simulink library "library_plc2simulink"  (R2017b)
settings: Solver=VariableStepAuto  StartTime=0.0  StopTime=10.0  RelTol=1e-3
libraries: simulink x2
settings Model: Creator=Moritz  LastModifiedBy=Moritz
settings DataIOCC: ReturnWorkspaceOutputs=on
settings SFSimCC: SimUseLocalCustomCode=on
settings RTWCC: RTWUseLocalCustomCode=on

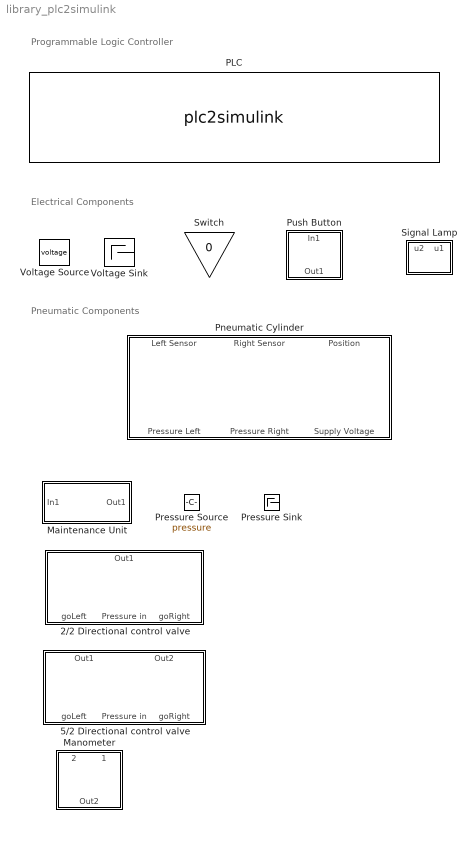
== system library_plc2simulink ==
  note: Programmable Logic Controller
  note: Electrical Components
  note: Pneumatic Components
  2/2 Directional control valve : Subsystem  mask{updateIcon=0.1, state=0}
      mask prompts: updateIcon "Icon Update Time (s):"
      mask init:
      | set_param(gcb,'MaskHideContents','on');
      mask Display:
      | stateValue = strcmpi(get_param(gcb(), 'state'), '1');
      | bigBlockWidth = 0.25;
      | smallBlockWidth = 0.1;
      | 
      | top = 0.85;
      | bottom = 0.3;
      | middle = bottom+(top-bottom)/2;
      | 
      | if ~stateValue
      |     x0=0;
      | else
      |     x0=bigBlockWidth;
      | end
      | 
      | %B1
      | plot(x0+smallBlockWidth*[0,0,1,1,0],[bottom,middle,middle,bottom,bottom]);
      | plot(x0+smallBlockWidth*[1/5,4/5], [bottom, middle]);
      | %B2
      | plot(x0+smallBlockWidth+bigBlockWidth*[0,0,1,1,0],[bottom,top,top,bottom,bottom]);
      | plot(x0+smallBlockWidth+bigBlockWidth*0.5*ones(1,2), [bottom, top]);
      | patch(x0+smallBlockWidth+bigBlockWidth*[0.4,0.5,0.6], top-(top-bottom)/5*[1,0,1]);
      | 
      | %B3
      | plot(x0+smallBlockWidth+bigBlockWidth+bigBlockWidth*[0,0,1,1,0],[bottom,top,top,bottom,bottom]);
      | plot(x0+smallBlockWidth+bigBlockWidth+bigBlockWidth*0.5*ones(1,2), [bottom, bottom+(top-bottom)/5]);
      | plot(x0+smallBlockWidth+bigBlockWidth+bigBlockWidth*0.5*ones(1,2), [top, top-(top-bottom)/5]);
      | plot(x0+smallBlockWidth+bigBlockWidth+bigBlockWidth*0.5+bigBlockWidth/8*[-1,1], top-(top-bottom)/5*ones(1,2));
      | plot(x0+smallBlockWidth+bigBlockWidth+bigBlockWidth*0.5+bigBlockWidth/8*[-1,1], bottom+(top-bottom)/5*ones(1,2));
      | 
      | %B4
      | plot(x0+smallBlockWidth+2*bigBlockWidth+smallBlockWidth*[0,0,1,1,0],[bottom,middle,middle,bottom,bottom]);
      | plot(x0+smallBlockWidth+2*bigBlockWidth+smallBlockWidth*[4/5,1/5], [bottom, middle]);
      | 
      | % Ports
      | port_label('input', 1, 'Ma');
      | port_label('input', 3, 'Mb');
      | 
      | % port connections
      | blockPos = get_param(gcb, 'Position');
      | blockWidthAbs = blockPos(3)-blockPos(1);
      | blockPosXAbs = blockPos(1);
      | ports = get_param(gcb(), 'PortHandles');
      | 
      | pressureIn = ports.Inport(2);
      | pressureInPos = get_param(pressureIn, 'Position');
      | pressureInX = (pressureInPos(1)-blockPosXAbs)/blockWidthAbs;
      | plot(pressureInX*ones(1,2), [0,bottom/2]);
      | plot(smallBlockWidth+bigBlockWidth*1.5*ones(1,2), [bottom/2, bottom]);
      | plot([pressureInX,smallBlockWidth+bigBlockWidth*1.5], bottom/2*ones(1,2));
      | 
      | pressureOut1 = ports.Outport(1);
      | pressureOut1Pos = get_param(pressureOut1, 'Position');
      | pressureOut1X = (pressureOut1Pos(1)-blockPosXAbs)/blockWidthAbs;
      | plot(pressureOut1X*ones(1,2), [1,1-(1-top)/2]);
      | plot(smallBlockWidth+bigBlockWidth*1.5*ones(1,2), [top,1-(1-top)/2]);
      | plot([pressureOut1X,smallBlockWidth+bigBlockWidth*1.5], (1-(1-top)/2)*ones(1,2));
  5/2 Directional control valve : Subsystem  mask{updateIcon=0.1, state=0}
      mask prompts: updateIcon "Update Icon Time (s):"
      mask init:
      | set_param(gcb,'MaskHideContents','on');
      mask Display:
      | stateValue = strcmpi(get_param(gcb(), 'state'), '1');
      | bigBlockWidth = 0.25;
      | smallBlockWidth = 0.1;
      | 
      | top = 0.85;
      | bottom = 0.3;
      | middle = bottom+(top-bottom)/2;
      | 
      | if ~stateValue
      |     x0=0;
      | else
      |     x0=bigBlockWidth;
      | end
      | 
      | %B1
      | plot(x0+smallBlockWidth*[0,0,1,1,0],[bottom,middle,middle,bottom,bottom]);
      | plot(x0+smallBlockWidth*[1/5,4/5], [bottom, middle]);
      | %B2
      | plot(x0+smallBlockWidth+bigBlockWidth*[0,0,1,1,0],[bottom,top,top,bottom,bottom]);
      | plot(x0+smallBlockWidth+bigBlockWidth*[0.5,0.25], [bottom, top]);
      | patch(x0+smallBlockWidth+bigBlockWidth*[0.19,0.29,0.39], top-(top-bottom)/5*[1,0,1]);
      | plot(x0+smallBlockWidth+bigBlockWidth*[0.75,0.75], [bottom, top]);
      | patch(x0+smallBlockWidth+bigBlockWidth*[0.65,0.75,0.85], bottom+(top-bottom)/5*[1,0,1]);
      | plot(x0+smallBlockWidth+bigBlockWidth*0.25*ones(1,2), [bottom, bottom+(top-bottom)/5]);
      | plot(x0+smallBlockWidth+bigBlockWidth*0.25+bigBlockWidth/8*[-1,1], bottom+(top-bottom)/5*ones(1,2));
      | 
      | %B3
      | plot(x0+smallBlockWidth+bigBlockWidth+bigBlockWidth*[0,0,1,1,0],[bottom,top,top,bottom,bottom]);
      | plot(x0+smallBlockWidth+bigBlockWidth+bigBlockWidth*[0.5,0.75], [bottom, top]);
      | patch(x0+smallBlockWidth+bigBlockWidth+bigBlockWidth*[0.63,0.73,0.83], top-(top-bottom)/5*[1,0,1]);
      | plot(x0+smallBlockWidth+bigBlockWidth+bigBlockWidth*[0.25,0.25], [bottom, top]);
      | patch(x0+smallBlockWidth+bigBlockWidth+bigBlockWidth*[0.15,0.25,0.35], bottom+(top-bottom)/5*[1,0,1]);
      | plot(x0+smallBlockWidth+bigBlockWidth+bigBlockWidth*0.75*ones(1,2), [bottom, bottom+(top-bottom)/5]);
      | plot(x0+smallBlockWidth+bigBlockWidth+bigBlockWidth*0.75+bigBlockWidth/8*[-1,1], bottom+(top-bottom)/5*ones(1,2));
      | 
      | %B4
      | plot(x0+smallBlockWidth+2*bigBlockWidth+smallBlockWidth*[0,0,1,1,0],[bottom,middle,middle,bottom,bottom]);
      | plot(x0+smallBlockWidth+2*bigBlockWidth+smallBlockWidth*[4/5,1/5], [bottom, middle]);
      | 
      | % ventiles
      | plot(smallBlockWidth+bigBlockWidth+bigBlockWidth*0.25+bigBlockWidth/8*[-1,0,1], [bottom, bottom-0.1,bottom])
      | plot(smallBlockWidth+bigBlockWidth+bigBlockWidth*0.75+bigBlockWidth/8*[-1,0,1], [bottom, bottom-0.1,bottom])
      | 
      | % Port labels
      | port_label('input', 1, 'Ma');
      | port_label('input', 3, 'Mb');
      | 
      | % port connections
      | blockPos = get_param(gcb, 'Position');
      | blockWidthAbs = blockPos(3)-blockPos(1);
      | blockPosXAbs = blockPos(1);
      | ports = get_param(gcb(), 'PortHandles');
      | 
      | pressureIn = ports.Inport(2);
      | pressureInPos = get_param(pressureIn, 'Position');
      | pressureInX = (pressureInPos(1)-blockPosXAbs)/blockWidthAbs;
      | plot(pressureInX*ones(1,2), [0,bottom/2]);
      | plot(smallBlockWidth+bigBlockWidth*1.5*ones(1,2), [bottom/2, bottom]);
      | plot([pressureInX,smallBlockWidth+bigBlockWidth*1.5], bottom/2*ones(1,2));
      | 
      | pressureOut1 = ports.Outport(1);
      | pressureOut1Pos = get_param(pressureOut1, 'Position');
      | pressureOut1X = (pressureOut1Pos(1)-blockPosXAbs)/blockWidthAbs;
      | plot(pressureOut1X*ones(1,2), [1,1-(1-top)/2]);
      | plot(smallBlockWidth+bigBlockWidth*1.25*ones(1,2), [top,1-(1-top)/2]);
      | plot([pressureOut1X,smallBlockWidth+bigBlockWidth*1.25], (1-(1-top)/2)*ones(1,2));
      | 
      | pressureOut2 = ports.Outport(2);
      | pressureOut2Pos = get_param(pressureOut2, 'Position');
      | pressureOut2X = (pressureOut2Pos(1)-blockPosXAbs)/blockWidthAbs;
      | plot(pressureOut2X*ones(1,2), [1,1-(1-top)/2]);
      | plot(smallBlockWidth+bigBlockWidth*1.75*ones(1,2), [top,1-(1-top)/2]);
      | plot([pressureOut2X,smallBlockWidth+bigBlockWidth*1.75], (1-(1-top)/2)*ones(1,2));
  Maintenance Unit : Subsystem  mask{pressure=1}
      mask prompts: pressure "Pressure (MPa):"
      mask init:
      | set_param(gcb,'MaskHideContents','on');
      mask DialogControl DescGroupVar Prompt: Maintenance Unit
      mask DialogControl DescTextVar Prompt: A pneumatic maintenance unit.
      mask Display:
      | % Get block parameters
      | pos = get_param(gcb, 'Position');
      | width = pos(3)-pos(1);
      | height = pos(4)-pos(2);
      | 
      | % plot box
      | plot([1,1,width-1,width-1,1,1], [1,height-1,height-1,1,1,height-1]);
      | 
      | % plot circle
      | radius = min(floor([width*2/5, height*2/5]))-1;
      | x = floor(width/2  + radius*sin(0:2*pi/50:2*pi));
      | y = floor(height/2 + radius*cos(0:2*pi/50:2*pi));
      | plot(x,y);
      | % plot arrow
      | arrowOuterRadius = 0.7*radius;
      | arrowInnerRadius = 0.2*radius;
      | dPi = pi/4;
      | plot(floor(width/2+arrowOuterRadius*sin(pi/4)*[1,-1]), floor(height/2+arrowOuterRadius*sin(pi/4)*[-1,1]));
      | patch(floor(width/2-[arrowOuterRadius*sin(pi/4),...
      |     arrowInnerRadius*sin(pi/4+dPi),...
      |     arrowInnerRadius*sin(pi/4-dPi)]),...
      |     floor(height/2+[arrowOuterRadius*cos(pi/4),...
      |     arrowInnerRadius*cos(pi/4+dPi),...
      |     arrowInnerRadius*cos(pi/4-dPi)]));
      | 
      | % plot filter
      | borderDash = 0.35;
      | numDash = 4;
      | dashHeight = (height-2)/(numDash+(numDash-1)*borderDash);
      | for i=0:numDash-1
      |     lineStart = 1 + i * dashHeight * (1+borderDash);
      |     plot(width/8*ones(1,2), [lineStart, lineStart+dashHeight]);
      | end
      | plot(width*7/8*ones(1,2), [height*3/4, height-1]);
  "Manometer " : Subsystem  mask{stateOn=0, updateIcon=0.1, actPressure=0.3}
      mask prompts: stateOn "State"; updateIcon "Icon Update Time (s):"; actPressure "Activation Pressure (MPa):"
      mask init:
      | set_param(gcb,'MaskHideContents','on');
      mask DialogControl DescGroupVar Prompt: Manometer
      mask DialogControl DescTextVar Prompt: Electrical contact is closed when pressure exceeds activation pressure.
      mask Display:
      | % Get block parameters
      | active = str2double(get_param(gcb, 'StateOn')) ~= 0;
      | pos = get_param(gcb, 'Position');
      | width = pos(3)-pos(1);
      | height = pos(4)-pos(2);
      | y0Abs = pos(1);
      | ports = get_param(gcb(), 'PortHandles');
      | pressureIn = ports.Inport(1);
      | pressureInPos = get_param(pressureIn, 'Position');
      | pressureInX = (pressureInPos(1)-y0Abs)/width;
      | powerIn = ports.Inport(2);
      | powerInPos = get_param(powerIn, 'Position');
      | powerInY = (powerInPos(1)-y0Abs)/width;
      | powerOut = ports.Outport(1);
      | powerOutPos = get_param(powerOut, 'Position');
      | powerOutY = (powerOutPos(1)-y0Abs)/width;
      | 
      | radius = 0.5;
      | xStart =radius/2;
      | xEnd = 1-radius/2;
      | yStart =  powerInY;
      | yEnd = height;
      | plot([0,xStart], powerInY*ones(1,2))
      | plot([xEnd,0.95], powerInY*ones(1,2))
      | plot(0.95*ones(1,2), [powerInY,powerOutY]);
      | plot([0.95,1], powerOutY*ones(1,2))
      | lineX = 1/2;
      | if active
      |     plot([xStart,xEnd+0.02], [yStart,yStart+radius/6]);
      |     plot(xEnd*ones(1,2), [yStart, yStart+radius/6+0.02])
      |     lineYStart = yStart+radius/12;
      |     lineYEnd = pressureInX;
      | else
      |     plot([xStart,xEnd], [yStart,yStart+radius/2]);
      |     lineYStart = yStart+radius/4;
      |     lineYEnd = pressureInX;
      | end
      | 
      | color('blue')
      | borderDash = 0.35;
      | numDash = 3;
      | dashHeight = (lineYEnd-lineYStart)/(numDash+(numDash-1)*borderDash);
      | for i=0:numDash-1
      |     lineStart = lineYStart + i * dashHeight * (1+borderDash);
      |     plot(lineX*ones(1,2), [lineStart, lineStart+dashHeight]);
      | end
      | borderDash = 0.35;
      | numDash = 3;
      | dashHeight = (lineX-0)/(numDash+(numDash-1)*borderDash);
      | for i=0:numDash-1
      |     lineStart = 0 + i * dashHeight * (1+borderDash);
      |     plot([lineStart, lineStart+dashHeight],lineYEnd*ones(1,2));
      | end
      | %port_label('input', 1, 'P')
  PLC : S-Function  FunctionName=plc2simulink  Parameters=instanceName, supplyVoltage,numInputs, numOutputs, timeStep,1  SFunctionDeploymentMode=off  EnableBusSupport=off  mask{instanceName=PLC1, numInputs=8, numOutputs=8, timeStep=0.05, externalSupplyVoltage=on}
      mask prompts: instanceName "PLC Instance Name"; numInputs "Number of Inputs:"; numOutputs "Number of Outputs:"; timeStep "Communication Update Time (s):"; externalSupplyVoltage "External Supply Voltage"
      mask init:
      | % Process parameters
      | if strcmpi(externalSupplyVoltage, 'on')
      |     supplyVoltage = 1.0;
      | else
      |     supplyVoltage = 0.0;
      | end
      | 
      | % Update SPS block
      | Simulink.Block.eval(gcb());
      mask DialogControl DescGroupVar Prompt: PLC Connection
      mask DialogControl DescTextVar Prompt: Connection to a PLC simulated via PLCSim Advanced.
      mask Display:
      | % Get parameters
      | numInputs = str2num(get_param(gcb(), 'numInputs'));
      | numOutputs = str2num(get_param(gcb(), 'numOutputs'));
      | externalSupplyVoltage = strcmpi(get_param(gcb(), 'externalSupplyVoltage'), 'on');
      | orientationParam = get_param(gcb,'Orientation');
      | rotated = strcmpi(orientationParam, 'up') || strcmpi(orientationParam, 'down');
      | instanceName = get_param(gcb,'instanceName');
      | 
      | % Set input port labels
      | if externalSupplyVoltage
      |     port_label('input',1,'L+');
      | end
      | for i=1:numInputs
      |     if externalSupplyVoltage
      |         idx = i+1;
      |     else
      |         idx = i;
      |     end
      |     port_label('input',idx,sprintf('I%g.%g', floor((i-1)/8), mod((i-1),8)))
      | end
      | 
      | % Set output port labels
      | if externalSupplyVoltage
      |     port_label('output',1,'L0');
      | end
      | for i=1:numOutputs
      |     if externalSupplyVoltage
      |         idx = i+1;
      |     else
      |         idx = i;
      |     end
      |     port_label('output',idx,sprintf('Q%g.%g', floor((i-1)/8), mod((i-1),8)))
      | end
      | % paint icon
      | %plot([0,1,1,0,0], [0,0,1,1,0]);
      | if ~rotated
      |     plot(0.25*ones(1,2), [0,1])
      |     plot(0.75*ones(1,2), [0,1])
      | else
      |     plot([0,1], 0.3*ones(1,2))
      |     plot([0,1], 0.7*ones(1,2))
      | end
      | text(0.5,0.5, instanceName, 'horizontalAlignment', 'center', 'verticalAlignment', 'middle');
  Pneumatic Cylinder : Subsystem  mask{minPos=0, maxPos=100, pistonSpeed=5, currentPos=0, updateIcon=0.1}
      mask prompts: minPos "Minimal Position (cm):"; maxPos "Maximal Position (cm):"; pistonSpeed "Piston Speed (cm/s/MPa):"; currentPos "Position (cm):"; updateIcon "Update Icon (s):"
      mask init:
      | set_param(gcb,'MaskHideContents','on');
      mask DialogControl DescGroupVar Prompt: Double-acting cylinder
      mask DialogControl DescTextVar Prompt: A double acting pneumatic cylinder.
      mask Display:
      | % Calculate relative position of piston
      | pos = str2double(get_param(gcb(), 'currentPos'));
      | maxPos = str2double(get_param(gcb(), 'maxPos'));
      | minPos = str2double(get_param(gcb(), 'minPos'));
      | relPos = (pos-minPos)/(maxPos-minPos);
      | 
      | % y-coordinates of drawn elements
      | bottomWall = 0.1;
      | wallHeight = 0.65;
      | pistonSmallBlockHeight = 0.4;
      | stickHeight = 0.16;
      | magnetHeight = 0.36;
      | magnetInnerHeight = 0.16;
      | 
      | topWall = bottomWall+wallHeight;
      | pistonSmallBlockBottom = bottomWall+(wallHeight-pistonSmallBlockHeight)/2;
      | pistonSmallBlockTop = pistonSmallBlockBottom+pistonSmallBlockHeight;
      | stickBottom = bottomWall+(wallHeight-stickHeight)/2;
      | stickTop = stickBottom+stickHeight;
      | magnetBottom = bottomWall+(wallHeight-magnetHeight)/2;
      | magnetTop = magnetBottom+magnetHeight;
      | magnetInnerBottom = bottomWall+(wallHeight-magnetInnerHeight)/2;
      | magnetInnerTop = magnetInnerBottom+magnetInnerHeight;
      | 
      | % x coordinate of drawn elements
      | stickWidth = 0.45;
      | pistonMainBlockWidth = 0.1;
      | pistonSmallBlockWidth = 0.03;
      | wallMargin = 0.015;
      | leftWall = 0;
      | pistonXMin = leftWall+wallMargin;
      | pistonXMax = 1-(pistonMainBlockWidth + 2*pistonSmallBlockWidth+stickWidth);
      | pistonX = relPos * (pistonXMax-pistonXMin)+pistonXMin;
      | rightWall = pistonXMax + pistonMainBlockWidth + 2*pistonSmallBlockWidth+wallMargin;
      | 
      | 
      | % Wall
      | plot(leftWall*ones(1,2), [bottomWall,topWall]);
      | plot([leftWall,rightWall], bottomWall*ones(1,2));
      | plot([leftWall,rightWall], topWall*ones(1,2));
      | plot(rightWall*ones(1,2), [bottomWall,stickBottom]);
      | plot(rightWall*ones(1,2), [stickTop,topWall]);
      | % piston block
      | plot(pistonX+[0,pistonSmallBlockWidth, pistonSmallBlockWidth, 0, 0], [pistonSmallBlockBottom,pistonSmallBlockBottom,pistonSmallBlockTop,pistonSmallBlockTop, pistonSmallBlockBottom]);
      | plot(pistonX+pistonSmallBlockWidth+[0,pistonMainBlockWidth, pistonMainBlockWidth, 0, 0], [bottomWall,bottomWall,topWall,topWall, bottomWall]);
      | plot(pistonX+pistonSmallBlockWidth+pistonMainBlockWidth+[0,pistonSmallBlockWidth, pistonSmallBlockWidth, 0, 0], [pistonSmallBlockBottom,pistonSmallBlockBottom,pistonSmallBlockTop,pistonSmallBlockTop, pistonSmallBlockBottom]);
      | % magnet
      | quarter = pistonMainBlockWidth/4;
      | patch(pistonX+pistonSmallBlockWidth+quarter+quarter*[0, 2,2,1,1,2,2,0],[magnetTop,magnetTop,magnetInnerTop,magnetInnerTop,magnetInnerBottom,magnetInnerBottom,magnetBottom,magnetBottom])
      | % stick
      | plot(pistonX+2*pistonSmallBlockWidth+pistonMainBlockWidth+[0,stickWidth, stickWidth, 0, 0], [stickBottom,stickBottom,stickTop,stickTop, stickBottom]);
      | 
      | % ports
      | port_label('input', 3, 'L+');
      | port_label('output', 1, 'BGa');
      | port_label('output', 2, 'BGb');
      | port_label('output', 3, 'pos');
      | 
      | % port connections
      | blockPos = get_param(gcb, 'Position');
      | blockWidthAbs = blockPos(3)-blockPos(1);
      | blockPosXAbs = blockPos(1);
      | ports = get_param(gcb(), 'PortHandles');
      | 
      | pressureIn1 = ports.Inport(1);
      | pressureInPos1 = get_param(pressureIn1, 'Position');
      | pressureInX1 = (pressureInPos1(1)-blockPosXAbs)/blockWidthAbs;
      | plot(pressureInX1*ones(1,2), [0,bottomWall/2]);
      | plot((leftWall+2*wallMargin)*ones(1,2), [bottomWall/2, bottomWall]);
      | plot([pressureInX1,leftWall+2*wallMargin], bottomWall/2*ones(1,2));
      | 
      | pressureIn2 = ports.Inport(2);
      | pressureInPos2 = get_param(pressureIn2, 'Position');
      | pressureInX1 = (pressureInPos2(1)-blockPosXAbs)/blockWidthAbs;
      | plot(pressureInX1*ones(1,2), [0,bottomWall/2]);
      | plot((rightWall-2*wallMargin)*ones(1,2), [bottomWall/2, bottomWall]);
      | plot([pressureInX1,rightWall-2*wallMargin], bottomWall/2*ones(1,2));
  Pressure Sink : Terminator
      mask Display: plot([0,1,1,0],[0.5,0,1,0.5]);
  Pressure Source : Constant  Value=pressure  mask{pressure=5}
      mask prompts: pressure "Pressure (MPa):"
      mask DialogControl DescGroupVar Prompt: Pressure Source
      mask DialogControl DescTextVar Prompt: Pneumatic pressure source.
      mask Display: plot([1,0,0,1],[0.5,0,1,0.5]);
  Push Button : Subsystem  mask{deactTime=1, StateOn=0}
      mask prompts: deactTime "Time until automatic deactivation (s):"; StateOn "State (0/1):"
      mask init:
      | set_param(gcb,'MaskHideContents','on');
      settings: OpenFcn=|
      | if str2double(get_param(gcb, 'StateOn')) ==0
      |   set_param(gcb, 'StateOn', '1');
      | end
      mask Display:
      | % Get block parameters
      | active = str2double(get_param(gcb, 'StateOn')) ~= 0;
      | pos = get_param(gcb, 'Position');
      | width = pos(3)-pos(1);
      | height = pos(4)-pos(2);
      | radius = min(floor(height/2), width-4);
      | 
      | xStart = floor((width-radius)/2);
      | xEnd = ceil(width-(width-radius)/2);
      | yStart = floor(height/2);
      | yEnd = height;
      | 
      | plot([0,xStart], yStart*ones(1,2))
      | plot([xEnd,width], yStart*ones(1,2))
      | 
      | lineX = floor(width/2);
      | if active
      |     plot([xStart,xEnd+2], [yStart,yStart+floor(radius/6)]);
      |     plot(xEnd*ones(1,2), [yStart, yStart+floor(radius/6)+2])
      |     lineYStart = yStart+floor(radius/12);
      |     lineYEnd = height-floor(radius/4);
      | else
      |     plot([xStart,xEnd], [yStart,yStart+floor(radius/2)]);
      |     lineYStart = yStart+floor(radius/4);
      |     lineYEnd = height;
      | end
      | 
      | borderDash = 0.35;
      | numDash = 3;
      | dashHeight = (lineYEnd-lineYStart)/(numDash+(numDash-1)*borderDash);
      | for i=0:numDash-1
      |     lineStart = lineYStart + i * dashHeight * (1+borderDash);
      |     plot(lineX*ones(1,2), [lineStart, lineStart+dashHeight]);
      | end
      | plot(lineX+ceil(dashHeight/2)*[-1,1], lineYEnd*ones(1,2));
  Signal Lamp : Subsystem  mask{Value=off, updateTime=0.1, colorOn=[0.2,1,0.2], colorOff=[1,1,1]}
      mask prompts: Value "State:"; updateTime "Update Time (s):"; colorOn "Color when ON:"; colorOff "Color when OFF:"
      mask init:
      | set_param(gcb,'MaskHideContents','on')
      mask TypeOptions Value: off | on
      mask DialogControl DescGroupVar Prompt: Signal Lamp
      mask DialogControl DescTextVar Prompt: Signal lamp which switches to ON if its two inputs are different.
      mask Display:
      | % Get block parameters
      | pos = get_param(gcb, 'Position');
      | width = pos(3)-pos(1);
      | height = pos(4)-pos(2);
      | radius = min(floor([width/2, height/2]))-1;
      | 
      | x = floor(width/2  + radius*sin(0:2*pi/50:2*pi));
      | y = floor(height/2 + radius*cos(0:2*pi/50:2*pi));
      | 
      | if strcmpi(get_param(gcb, 'Value'), 'on');
      |     colorLight = eval(get_param(gcb, 'colorOn'));
      | else
      |     colorLight = eval(get_param(gcb, 'colorOff'));
      | end
      | patch(x,y, colorLight);
      | color('black');
      | plot(x-1,y);
      | xStart = 0.5-0.45*sin(pi/4);
      | plot(floor(width/2+radius*sin(pi/4)*[1,-1]), floor(height/2+radius*sin(pi/4)*[1,-1]));
      | plot(floor(width/2+radius*sin(pi/4)*[1,-1]), floor(height/2+radius*sin(pi/4)*[-1,1]));
      | return;
  Switch : Gain  Gain=0
      settings: OpenFcn=|
      | if str2double(get_param(gcb, 'Gain')) ~=0
      |   set_param(gcb, 'Gain', '0');
      | else
      |   set_param(gcb, 'Gain', '1');
      | end
      mask Display:
      | % Get block parameters
      | active = str2double(get_param(gcb, 'Gain')) ~= 0;
      | pos = get_param(gcb, 'Position');
      | width = pos(3)-pos(1);
      | height = pos(4)-pos(2);
      | radius = min(floor(height/2), width-4);
      | 
      | xStart = floor((width-radius)/2);
      | xEnd = ceil(width-(width-radius)/2);
      | yStart = floor(height/2);
      | yEnd = height;
      | 
      | plot([0,xStart], yStart*ones(1,2))
      | plot([xEnd,width], yStart*ones(1,2))
      | 
      | lineX = floor(width/2);
      | if active
      |     plot([xStart,xEnd+2], [yStart,yStart+floor(radius/6)]);
      |     plot(xEnd*ones(1,2), [yStart, yStart+floor(radius/6)+2])
      |     lineYStart = yStart+floor(radius/12);
      |     lineYEnd = height-floor(radius/4);
      | else
      |     plot([xStart,xEnd], [yStart,yStart+floor(radius/2)]);
      |     lineYStart = yStart+floor(radius/4);
      |     lineYEnd = height;
      | end
      | 
      | borderDash = 0.35;
      | numDash = 3;
      | dashHeight = (lineYEnd-lineYStart)/(numDash+(numDash-1)*borderDash);
      | for i=0:numDash-1
      |     lineStart = lineYStart + i * dashHeight * (1+borderDash);
      |     if i == (numDash-1)/2
      |         plot(lineX-[0,0,floor(dashHeight),0,0], [lineStart, lineStart,lineStart+floor(dashHeight/2), lineStart+dashHeight,lineStart+dashHeight]);
      |     else
      |         plot(lineX*ones(1,2), [lineStart, lineStart+dashHeight]);
      |     end
      | end
      | plot(lineX+ceil(dashHeight/2)*[-1,1], lineYEnd*ones(1,2));
  Voltage Sink : Terminator
      mask DialogControl DescGroupVar Prompt: Voltage Sink
      mask Display:
      | x = 0.5+0.1*sin(0:0.1:2*pi);
      | y = 0.5+0.1*cos(0:0.1:2*pi);
      | plot(x,y);
      | plot([0.4,0],[0.5,0.5])
      | 
      | text(0.5,0.6, '0V', 'horizontalAlignment', 'center', 'verticalAlignment', 'bottom')
  Voltage Source : Constant  Value=voltage  mask{voltage=24}
      mask prompts: voltage "Voltage (V):"
      mask DialogControl DescGroupVar Prompt: Voltage Source
      mask Display:
      | value = get_param(gcb, 'voltage');
      | x = 0.5+0.1*sin(0:0.1:2*pi);
      | y = 0.5+0.1*cos(0:0.1:2*pi);
      | plot(x,y);
      | plot([0.6,1],[0.5,0.5])
      | 
      | text(0.5,0.6, [value,'V'], 'horizontalAlignment', 'center', 'verticalAlignment', 'bottom')

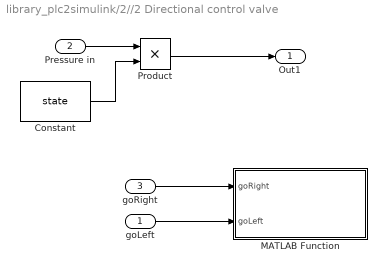
== system library_plc2simulink/2//2 Directional control valve ==
  goLeft : Inport
  Pressure in : Inport  Port=2
  goRight : Inport  Port=3
  Constant : Constant  Value=state
  MATLAB Function : MATLAB Function  TreatAsAtomicUnit=on  SystemSampleTime=updateIcon
  Product : Product
  Out1 : Outport
  wires:
  Constant/1 -> Product/2
  Pressure in/1 -> Product/1
  Product/1 -> Out1/1
  goRight/1 -> MATLAB Function/1(goRight)
  goLeft/1 -> MATLAB Function/2(goLeft)

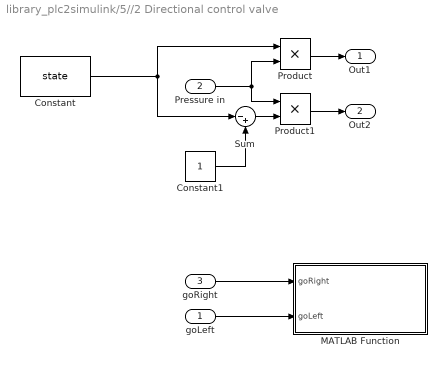
== system library_plc2simulink/5//2 Directional control valve ==
  goLeft : Inport
  Pressure in : Inport  Port=2
  goRight : Inport  Port=3
  Constant : Constant  Value=state
  Constant1 : Constant
  MATLAB Function : MATLAB Function  TreatAsAtomicUnit=on  SystemSampleTime=updateIcon
  Product : Product
  Product1 : Product
  Sum : Sum  Inputs=|-+
  Out1 : Outport
  Out2 : Outport  Port=2
  wires:
  goLeft/1 -> MATLAB Function/2(goLeft)
  goRight/1 -> MATLAB Function/1(goRight)
  Constant/1 -> Sum/1, Product/1
  Product/1 -> Out1/1
  Constant1/1 -> Sum/2
  Sum/1 -> Product1/2
  Product1/1 -> Out2/1
  Pressure in/1 -> Product1/1, Product/2

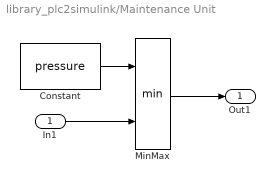
== system library_plc2simulink/Maintenance Unit ==
  In1 : Inport
  Constant : Constant  Value=pressure
  MinMax : MinMax  Inputs=2
  Out1 : Outport
  wires:
  Constant/1 -> MinMax/1
  In1/1 -> MinMax/2
  MinMax/1 -> Out1/1

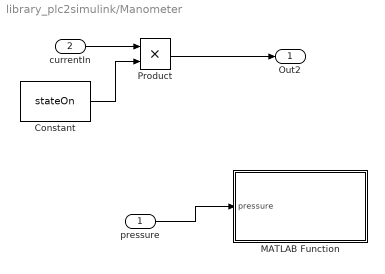
== system library_plc2simulink/Manometer  ==
  pressure : Inport
  currentIn : Inport  Port=2
  Constant : Constant  Value=stateOn
  MATLAB Function : MATLAB Function  TreatAsAtomicUnit=on  SystemSampleTime=updateIcon
  Product : Product
  Out2 : Outport
  wires:
  Constant/1 -> Product/2
  pressure/1 -> MATLAB Function/1(pressure)
  currentIn/1 -> Product/1
  Product/1 -> Out2/1

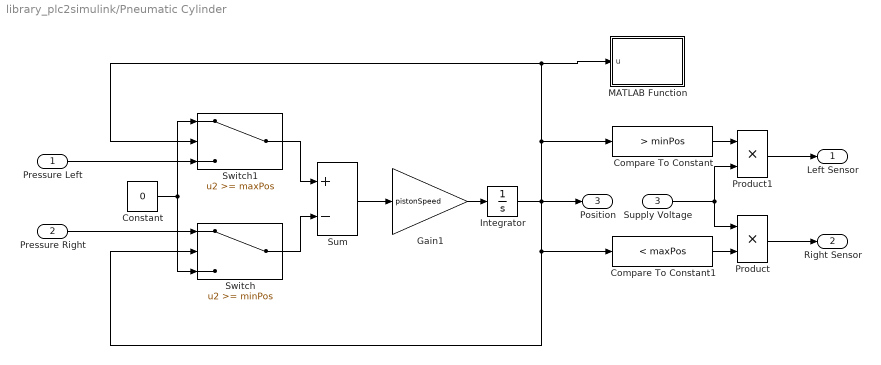
== system library_plc2simulink/Pneumatic Cylinder ==
  Pressure Left : Inport
  Pressure Right : Inport  Port=2
  Supply Voltage : Inport  Port=3
  Compare To Constant : simulink/Logic and Bit Operations/Compare To Constant  relop=>  const=minPos  OutDataTypeStr=boolean
  Compare To Constant1 : simulink/Logic and Bit Operations/Compare To Constant  relop=<  const=maxPos  OutDataTypeStr=boolean
  Constant : Constant  Value=0
  Gain1 : Gain  Gain=pistonSpeed
  Integrator : Integrator
  MATLAB Function : MATLAB Function  TreatAsAtomicUnit=on  SystemSampleTime=updateIcon
  Product : Product
  Product1 : Product
  Sum : Sum  Inputs=+-
  Switch : Switch  Threshold=minPos
  Switch1 : Switch  Threshold=maxPos
  Left Sensor : Outport
  Right Sensor : Outport  Port=2
  Position : Outport  Port=3
  wires:
  Product1/1 -> Left Sensor/1
  Compare To Constant/1 -> Product1/1
  Supply Voltage/1 -> Product1/2, Product/1
  Product/1 -> Right Sensor/1
  Compare To Constant1/1 -> Product/2
  Switch/1 -> Sum/2
  Switch1/1 -> Sum/1
  Sum/1 -> Gain1/1
  Constant/1 -> Switch1/1, Switch/3
  Pressure Left/1 -> Switch1/3
  Integrator/1 -> Compare To Constant/1, MATLAB Function/1(u), Switch1/2, Switch/2, Compare To Constant1/1, Position/1
  Pressure Right/1 -> Switch/1
  Gain1/1 -> Integrator/1

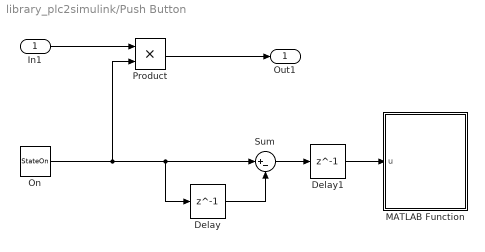
== system library_plc2simulink/Push Button ==
  In1 : Inport
  Delay : Delay  DelayLength=1  InitialCondition=0  SampleTime=deactTime
  Delay1 : Delay  DelayLength=1  InitialCondition=0  SampleTime=deactTime
  MATLAB Function : MATLAB Function  TreatAsAtomicUnit=on  SystemSampleTime=deactTime
  On : Constant  Value=StateOn
  Product : Product
  Sum : Sum  Inputs=|+-
  Out1 : Outport
  wires:
  On/1 -> Product/2, Delay/1, Sum/1
  Delay/1 -> Sum/2
  Product/1 -> Out1/1
  In1/1 -> Product/1
  Sum/1 -> Delay1/1
  Delay1/1 -> MATLAB Function/1(u)

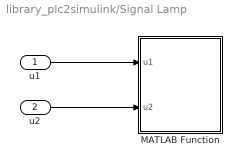
== system library_plc2simulink/Signal Lamp ==
  u1 : Inport
  u2 : Inport  Port=2
  MATLAB Function : MATLAB Function  TreatAsAtomicUnit=on
  wires:
  u1/1 -> MATLAB Function/1(u1)
  u2/1 -> MATLAB Function/2(u2)

== matlab function library_plc2simulink/Push Button/MATLAB Function ==
  data: u input
function updateState(u) %#eml

eml.extrinsic('set_param');
eml.extrinsic('get_param');
eml.extrinsic('gcb');

if u ~= 0
    parent = get_param(gcb(), 'Parent');
    set_param(parent, 'StateOn', '0');
end
end

== matlab function library_plc2simulink/Signal Lamp/MATLAB Function ==
  data: u1 input; u2 input
function updateIcon(u1, u2) %#eml

eml.extrinsic('set_param');
eml.extrinsic('get_param');
eml.extrinsic('num2str');
eml.extrinsic('gcb');

parent = get_param(gcb(), 'Parent');
if u1 ~= u2
    if ~strcmpi(get_param(parent, 'Value'), 'on')
        set_param(parent, 'Value', 'on');
    end
else
    if ~strcmpi(get_param(parent, 'Value'), 'off')
        set_param(parent, 'Value', 'off');
    end
end
end

== matlab function library_plc2simulink/Pneumatic Cylinder/MATLAB Function ==
  data: u input
function updateIcon(u) %#eml

eml.extrinsic('set_param');
eml.extrinsic('get_param');
eml.extrinsic('num2str');
eml.extrinsic('str2double');
eml.extrinsic('gcb');

parent = get_param(gcb(), 'Parent');
val = num2str(u);
if ~strcmpi(get_param(parent, 'currentPos'), val)
    set_param(parent, 'currentPos', val);
end
end

== matlab function library_plc2simulink/2//2 Directional control valve/MATLAB Function ==
  data: goRight input; goLeft input
function updateIcon(goRight, goLeft) %#eml

eml.extrinsic('set_param');
eml.extrinsic('get_param');
eml.extrinsic('num2str');
eml.extrinsic('str2double');
eml.extrinsic('gcb');

if goRight == goLeft
    return;
end

parent = get_param(gcb(), 'Parent');
if goRight > goLeft
    if ~strcmpi(get_param(parent, 'state'), '0')
        set_param(parent, 'state', '0');
    end
elseif goLeft > goRight
    if ~strcmpi(get_param(parent, 'state'), '1')
        set_param(parent, 'state', '1');
    end
end
end

== matlab function library_plc2simulink/5//2 Directional control valve/MATLAB Function ==
  data: goRight input; goLeft input
function updateIcon(goRight, goLeft) %#eml

eml.extrinsic('set_param');
eml.extrinsic('get_param');
eml.extrinsic('num2str');
eml.extrinsic('str2double');
eml.extrinsic('gcb');

if goRight == goLeft
    return;
end

parent = get_param(gcb(), 'Parent');
if goRight > goLeft
    if ~strcmpi(get_param(parent, 'state'), '0')
        set_param(parent, 'state', '0');
    end
elseif goLeft > goRight
    if ~strcmpi(get_param(parent, 'state'), '1')
        set_param(parent, 'state', '1');
    end
end
end

== matlab function library_plc2simulink/Manometer /MATLAB Function ==
  data: pressure input
function updateIcon(pressure) %#eml

eml.extrinsic('set_param');
eml.extrinsic('get_param');
eml.extrinsic('num2str');
eml.extrinsic('str2double');
eml.extrinsic('gcb');
eml.extrinsic('gt');

parent = get_param(gcb(), 'Parent');
actPressure = str2double(get_param(parent, 'actPressure'));
if gt(pressure, actPressure)
    if ~strcmpi(get_param(parent, 'stateOn'), '1')
        set_param(parent, 'stateOn', '1');
    end
else
    if ~strcmpi(get_param(parent, 'stateOn'), '0')
        set_param(parent, 'stateOn', '0');
    end
end
end
